simulink model "threebanbo"  (R2023b)
settings: Solver=ode23tb  StartTime=0.0  StopTime=0.1  RelTol=1e-3
libraries: spsCurrentMeasurementLib x4, spsVoltageMeasurementLib x4, spsACVoltageSourceLib x3, spsThyristorLib x3, spsGroundLib x2, spsSeriesRLCBranchLib x1, sps_lib x1
settings Model: Creator=Administrator  LastModifiedBy=ASUS

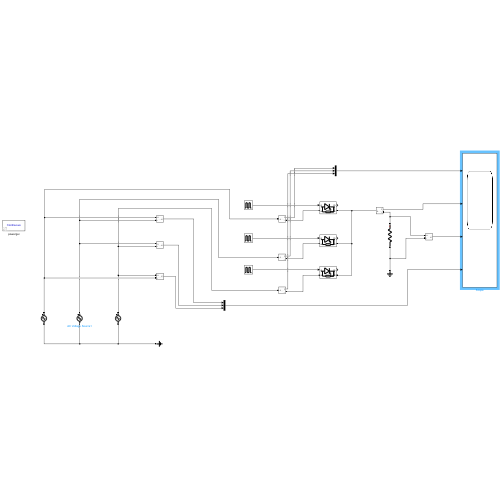
[thumbnail: Simulink's stored preview of the top-level diagram]
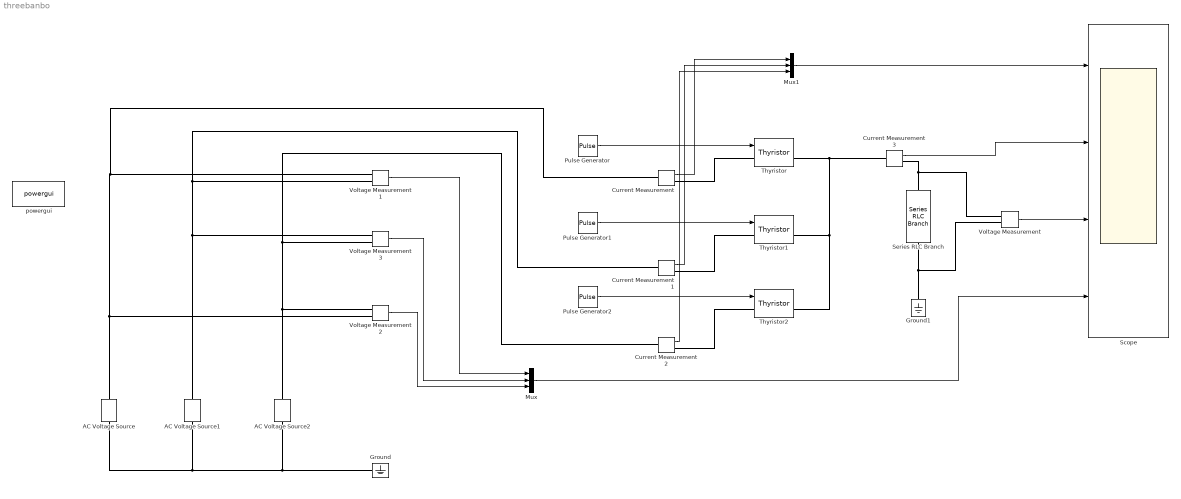
== system threebanbo ==
  AC Voltage Source : spsACVoltageSourceLib/AC Voltage Source  Amplitude=380  Phase=0  Frequency=50  SampleTime=0  Measurements=None  BusType=swing  Pref=10e3  Qref=0  Qmin=-inf  Qmax=+inf
  AC Voltage Source1 : spsACVoltageSourceLib/AC Voltage Source  Amplitude=380  Phase=-120  Frequency=50  SampleTime=0  Measurements=None  BusType=swing  Pref=10e3  Qref=0  Qmin=-inf  Qmax=+inf
  AC Voltage Source2 : spsACVoltageSourceLib/AC Voltage Source  Amplitude=380  Phase=-240  Frequency=50  SampleTime=0  Measurements=None  BusType=swing  Pref=10e3  Qref=0  Qmin=-inf  Qmax=+inf
  Current Measurement{,1..3} (4 alike) : spsCurrentMeasurementLib/Current Measurement  PhasorSimulation=off  OutputType=Complex  PSBequivalent=0
  Ground : spsGroundLib/Ground  LConnTagsString=a
  Ground1 : spsGroundLib/Ground  LConnTagsString=a
  Mux : Mux  Inputs=3
  Mux1 : Mux  Inputs=3
  Pulse Generator : DiscretePulseGenerator  PulseType=Time based  Amplitude=5  Period=0.02  PulseWidth=2  PhaseDelay=30*0.02/360
  Pulse Generator1 : DiscretePulseGenerator  PulseType=Time based  Amplitude=5  Period=0.02  PulseWidth=2  PhaseDelay=150*0.02/360
  Pulse Generator2 : DiscretePulseGenerator  PulseType=Time based  Amplitude=5  Period=0.02  PulseWidth=2  PhaseDelay=270*0.02/360
  Scope : Scope  NumInputPorts=4
  Series RLC Branch : spsSeriesRLCBranchLib/Series RLC Branch  LConnTagsString=__new0  RConnTagsString=__new0  BranchType=R  Resistance=1  Inductance=0  SetiL0=off  InitialCurrent=0  Capacitance=inf  Setx0=off  InitialVoltage=0  Measurements=None
  Thyristor : spsThyristorLib/Thyristor  Ron=0.001  Lon=0  Vf=0  IC=0  Rs=50  Cs=250e-9  Measurements=on
  Thyristor1 : spsThyristorLib/Thyristor  Ron=0.001  Lon=0  Vf=0  IC=0  Rs=50  Cs=250e-9  Measurements=on
  Thyristor2 : spsThyristorLib/Thyristor  Ron=0.001  Lon=0  Vf=0  IC=0  Rs=50  Cs=250e-9  Measurements=on
  Voltage Measurement{,1..3} (4 alike) : spsVoltageMeasurementLib/Voltage Measurement  PhasorSimulation=off  OutputType=Complex  PSBequivalent=0
  powergui : sps_lib/powergui  Priority=1  SimulationMode=Continuous  SampleTime=50e-6  frequency=60  Iterations=50  frequencyindice=50  Pbase=100e6  ErrMax=1e-4  UnitsV=kV  UnitsW=MW  buscounter=0  FunctionMessages=off  echomessages=off  EnableUseOfTLC=off  CurrentSourceSwitches=off  DisableSnubberDevices=off  DisableRonSwitches=off  DisableVfSwitches=off  DisplayEquations=off  AutomaticDiscreteSolvers=off  SolverType=Tustin/Backward Euler (TBE)  Interpol=off  ExternalGateDelay=off  methode=off  Ts=100  x0status=blocks  SPID=on  SwTol=0  HookPort=off  NonlinearTolerance=1e-4  nMaxIteration=100  ContinueOnMaxIteration=off  RestoreLinks=warning  ResistiveCurrentMeasurement=off  Frange=[0:2:500]  Ylog=off  Xlog=on  ShowGrid=off  save=off  variable=ZData  structure=0  ZoomFFT=off  StartTime=0.0  cycles=1  DisplayStyle=1  fundamental=60  FreqAxis=off  MaxFrequency=1000  frequencyindicesteady=1  RmsSteady=1  display=off
  wires:
  Voltage Measurement1/1 -> Mux/1
  Voltage Measurement3/1 -> Mux/2
  Voltage Measurement2/1 -> Mux/3
  Pulse Generator/1 -> Thyristor/1
  Pulse Generator1/1 -> Thyristor1/1
  Pulse Generator2/1 -> Thyristor2/1
  Current Measurement/1 -> Mux1/1
  Current Measurement1/1 -> Mux1/2
  Current Measurement2/1 -> Mux1/3
  Mux1/1 -> Scope/1
  Mux/1 -> Scope/4
  Current Measurement3/1 -> Scope/2
  Voltage Measurement/1 -> Scope/3
  connections:
  AC Voltage Source/LConn1 -- AC Voltage Source2/LConn1 -- Ground/LConn1 -- AC Voltage Source1/LConn1
  Voltage Measurement2/LConn2 -- Current Measurement/LConn1 -- Voltage Measurement1/LConn1 -- AC Voltage Source/RConn1
  AC Voltage Source2/RConn1 -- Current Measurement2/LConn1 -- Voltage Measurement3/LConn2 -- Voltage Measurement2/LConn1
  AC Voltage Source1/RConn1 -- Voltage Measurement3/LConn1 -- Current Measurement1/LConn1 -- Voltage Measurement1/LConn2
  Current Measurement/RConn1 -- Thyristor/LConn1
  Current Measurement1/RConn1 -- Thyristor1/LConn1
  Current Measurement2/RConn1 -- Thyristor2/LConn1
  Thyristor/RConn1 -- Thyristor2/RConn1 -- Thyristor1/RConn1 -- Current Measurement3/LConn1
  Current Measurement3/RConn1 -- Voltage Measurement/LConn1 -- Series RLC Branch/LConn1
  Series RLC Branch/RConn1 -- Voltage Measurement/LConn2 -- Ground1/LConn1
